simulink model "tcp_model"  (R2025b)
settings: Solver=FixedStepAuto  StartTime=0.0  StopTime=120  FixedStep=0.1  RelTol=1e-3

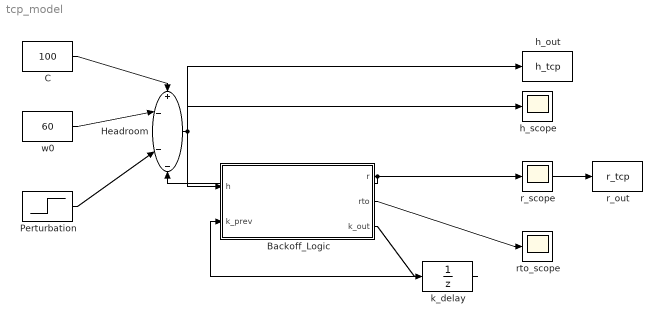
== system tcp_model ==
  Backoff_Logic : MATLAB Function  TreatAsAtomicUnit=on
  C : Constant  Value=100
  Headroom : Sum  Inputs=+---
  Perturbation : Step  Time=5  After=30  SampleTime=0
  h_out : ToWorkspace  VariableName=h_tcp  SaveFormat=Timeseries  SampleTime=-1
  h_scope : Scope
  k_delay : UnitDelay  SampleTime=0.1  HasFrameUpgradeWarning=on
  r_out : ToWorkspace  VariableName=r_tcp  SaveFormat=Timeseries  SampleTime=-1
  r_scope : Scope
  rto_scope : Scope
  w0 : Constant  Value=60
  wires:
  C/1 -> Headroom/1
  w0/1 -> Headroom/2
  Perturbation/1 -> Headroom/3
  Headroom/1 -> Backoff_Logic/1(h), h_scope/1, h_out/1
  k_delay/1 -> Backoff_Logic/2(k_prev)
  Backoff_Logic/1(r) -> Headroom/4, r_scope/1, r_out/1
  Backoff_Logic/3(k_out) -> k_delay/1
  Backoff_Logic/2(rto) -> rto_scope/1

== matlab function tcp_model/Backoff_Logic ==
  data: h input; r output; k_prev input; rto output; k_out output
function [r, rto, k_out] = Backoff_Logic(h, k_prev)
% Exponential backoff retransmission logic.
% h: current headroom (scalar)
% k_prev: previous timeout count
% r: retransmission rate (segments/RTT)
% rto: current RTO
% k_out: updated timeout count
RTO_base = 1;
max_retries = 15;
if h < 0 && k_prev < max_retries
    k_out = k_prev + 1;
elseif h >= 0 && k_prev > 0
    k_out = max(0, k_prev - 1);
else
    k_out = k_prev;
end
rto = RTO_base * 2^k_out;
if k_out > 0
    r = 1 / rto;
else
    r = 0;
end
